simulink model "ADRC_1RD_TEST"  (Simulink 7.6)
settings: Solver=ode45  StartTime=0.0  StopTime=500  RelTol=1e-3
values from neighbouring files (symbols this model uses):
  K = [9.375  -6.25; -8.125  8.75]    [PP2013428.mat]
libraries: ADRC x2
settings Model: Creator=Administrator  LastModifiedBy=Administrator
settings DebuggingCC: AlgebraicLoopMsg=none  ArtificialAlgebraicLoopMsg=none  SolverPrmCheckMsg=none  UnknownTsInhSupMsg=none

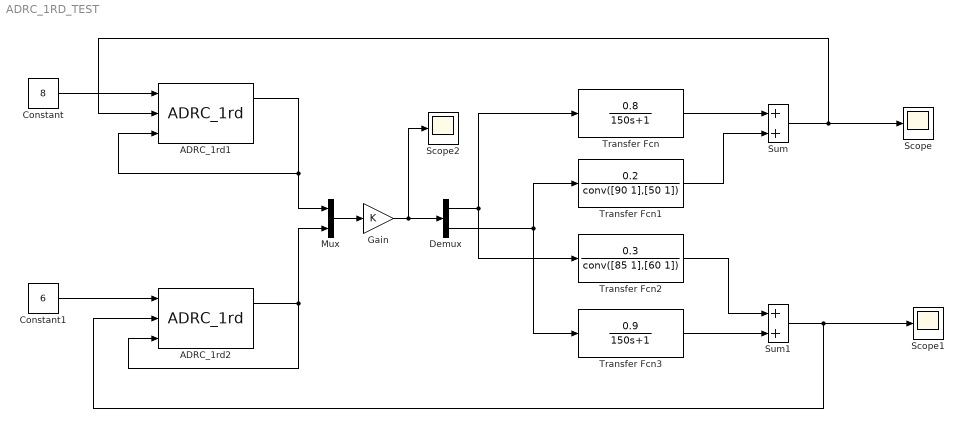
== system ADRC_1RD_TEST ==
  ADRC_1rd1 : ADRC/ADRC/ADRC_1rd/ADRC_1rd  SystemSampleTime=-1  r0=0.003  h=0.1  B01=10  B02=300  r=0.3
  ADRC_1rd2 : ADRC/ADRC/ADRC_1rd/ADRC_1rd  SystemSampleTime=-1  r0=0.003  h=0.1  B01=10  B02=300  r=0.3
  Constant : Constant  Value=8
  Constant1 : Constant  Value=6
  Demux : Demux  Outputs=2
  Gain : Gain  Gain=K
  Mux : Mux  Inputs=2
  Scope : Scope
      settings: TimeRange=500  YMin=7.9999  YMax=8.0002  DataFormat=Array
  Scope1 : Scope
      settings: TimeRange=500  YMin=7.9999  YMax=8.0002  DataFormat=Array
  Scope2 : Scope
      settings: TimeRange=500  YMin=7.9999  YMax=8.0002  SaveName=ScopeData2  DataFormat=Array
  Sum : Sum
  Sum1 : Sum
  Transfer Fcn : TransferFcn  Numerator=0.8  Denominator=[150 1]
  Transfer Fcn1 : TransferFcn  Numerator=0.2  Denominator=conv([90 1],[50 1])
  Transfer Fcn2 : TransferFcn  Numerator=0.3  Denominator=conv([85 1],[60 1])
  Transfer Fcn3 : TransferFcn  Numerator=0.9  Denominator=[150 1]
  wires:
  Constant/1 -> ADRC_1rd1/1
  Transfer Fcn/1 -> Sum/1
  Constant1/1 -> ADRC_1rd2/1
  Mux/1 -> Gain/1
  Gain/1 -> Demux/1, Scope2/1
  ADRC_1rd1/1 -> Mux/1, ADRC_1rd1/3
  ADRC_1rd2/1 -> Mux/2, ADRC_1rd2/3
  Transfer Fcn3/1 -> Sum1/2
  Demux/1 -> Transfer Fcn/1, Transfer Fcn2/1
  Demux/2 -> Transfer Fcn1/1, Transfer Fcn3/1
  Sum/1 -> ADRC_1rd1/2, Scope/1
  Transfer Fcn1/1 -> Sum/2
  Transfer Fcn2/1 -> Sum1/1
  Sum1/1 -> Scope1/1, ADRC_1rd2/2
